simulink model "simulink_sis_fis"  (R2024a)
settings: Solver=VariableStepAuto  StartTime=0.0  StopTime=10.0  RelTol=1e-3
InitFcn:
  | m1=290;
  | b1=1000;
  | m2=59;
  | k1=16182;
  | f=0;
  | k2=19000;

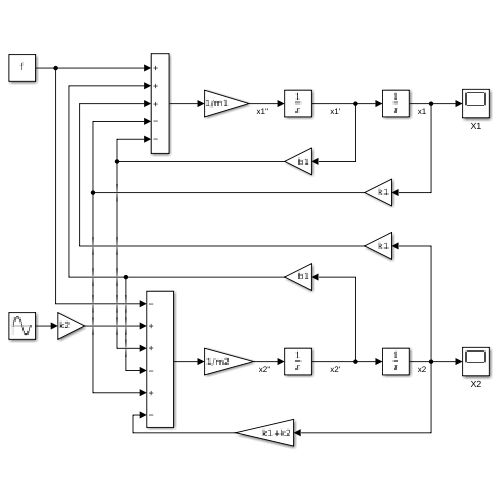
[thumbnail: Simulink's stored preview of the top-level diagram]
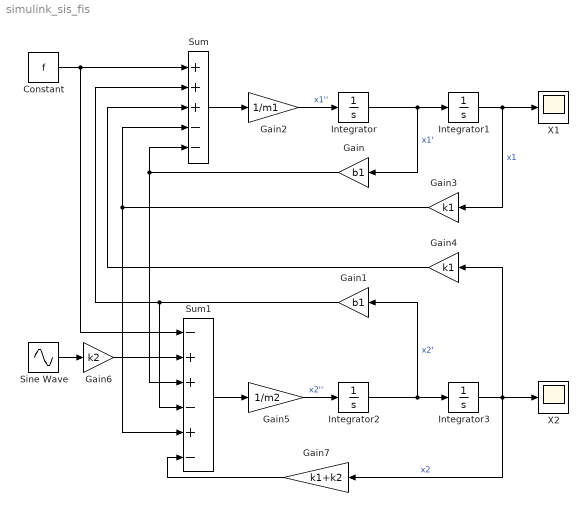
== system simulink_sis_fis ==
  Constant : Constant  Value=f
  Gain : Gain  Gain=b1
  Gain1 : Gain  Gain=b1
  Gain2 : Gain  Gain=1/m1
  Gain3 : Gain  Gain=k1
  Gain4 : Gain  Gain=k1
  Gain5 : Gain  Gain=1/m2
  Gain6 : Gain  Gain=k2
  Gain7 : Gain  Gain=k1+k2
  Integrator{,1..3} (4 alike) : Integrator
  Sine Wave : Sin  Amplitude=0.05  Frequency=0.5*pi  SampleTime=0
  Sum : Sum  Inputs=+++--
  Sum1 : Sum  Inputs=-++-+-
  X1 : Scope
  X2 : Scope
  wires:
  Integrator/1 -> Gain/1, Integrator1/1  "x1'"
  Integrator2/1 -> Integrator3/1, Gain1/1  "x2'"
  Sum/1 -> Gain2/1
  Gain2/1 -> Integrator/1  "x1''"
  Gain/1 -> Sum1/3, Sum/5
  Gain1/1 -> Sum1/4, Sum/2
  Integrator3/1 -> X2/1, Gain4/1, Gain7/1  "x2"
  Integrator1/1 -> X1/1, Gain3/1  "x1"
  Gain3/1 -> Sum1/5, Sum/4
  Gain4/1 -> Sum/3
  Sum1/1 -> Gain5/1
  Gain5/1 -> Integrator2/1  "x2''"
  Constant/1 -> Sum1/1, Sum/1
  Sine Wave/1 -> Gain6/1
  Gain6/1 -> Sum1/2
  Gain7/1 -> Sum1/6
